simulink model "class_09"  (R2023b)
settings: Solver=VariableStepAuto  StartTime=0.0  StopTime=10.0  RelTol=1e-3
libraries: cstblocks x10
settings Model: Creator=klysm  LastModifiedBy=klysm

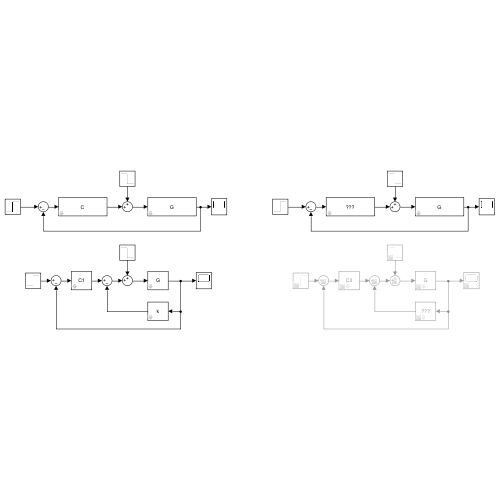
[thumbnail: Simulink's stored preview of the top-level diagram]
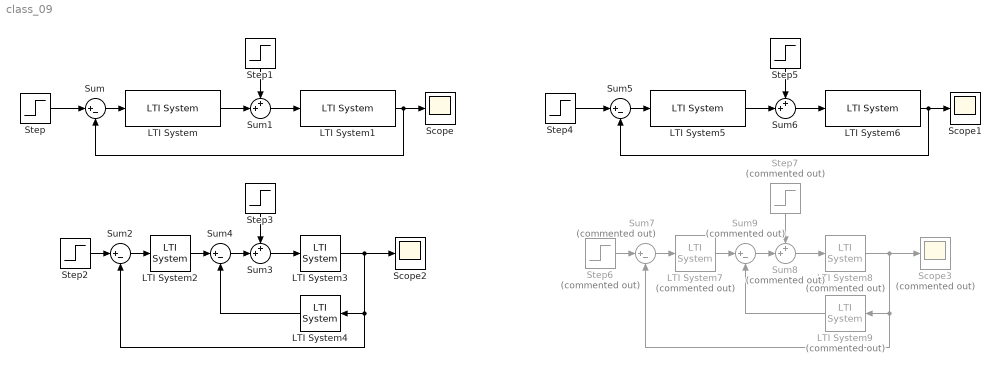
== system class_09 ==
  LTI System : cstblocks/LTI System  sys=C  IC=[]  PadeOrder=0
  LTI System1 : cstblocks/LTI System  sys=G  IC=[]  PadeOrder=0
  LTI System2 : cstblocks/LTI System  sys=C1  IC=[]  PadeOrder=0
  LTI System3 : cstblocks/LTI System  sys=G  IC=[]  PadeOrder=0
  LTI System4 : cstblocks/LTI System  sys=k  IC=[]  PadeOrder=0
  LTI System5 : cstblocks/LTI System  sys=C2  IC=[]  PadeOrder=0
  LTI System6 : cstblocks/LTI System  sys=G  IC=[]  PadeOrder=0
  LTI System7 : cstblocks/LTI System  Commented=on  sys=C3  IC=[]  PadeOrder=0
  LTI System8 : cstblocks/LTI System  Commented=on  sys=G  IC=[]  PadeOrder=0
  LTI System9 : cstblocks/LTI System  Commented=on  sys=C4  IC=[]  PadeOrder=0
  Scope : Scope
  Scope1 : Scope
  Scope2 : Scope
  Scope3 : Scope  Commented=on
  Step : Step  Time=0  SampleTime=0
  Step1 : Step  Time=5  After=-5  SampleTime=0
  Step2 : Step  Time=0  SampleTime=0
  Step3 : Step  Time=5  After=-5  SampleTime=0
  Step4 : Step  Time=0  SampleTime=0
  Step5 : Step  Time=5  After=-5  SampleTime=0
  Step6 : Step  Commented=on  Time=0  SampleTime=0
  Step7 : Step  Commented=on  Time=5  After=-5  SampleTime=0
  Sum{,2,4..5} (4 alike) : Sum  Inputs=|+-
  Sum1 : Sum  Inputs=++|
  Sum3 : Sum  Inputs=++|
  Sum6 : Sum  Inputs=++|
  Sum7 : Sum  Commented=on  Inputs=|+-
  Sum8 : Sum  Commented=on  Inputs=++|
  Sum9 : Sum  Commented=on  Inputs=|+-
  wires:
  LTI System/1 -> Sum1/2
  LTI System1/1 -> Sum/2, Scope/1
  Step/1 -> Sum/1
  Sum/1 -> LTI System/1
  Sum1/1 -> LTI System1/1
  Step1/1 -> Sum1/1
  Sum3/1 -> LTI System3/1
  Sum2/1 -> LTI System2/1
  Step3/1 -> Sum3/1
  LTI System3/1 -> Scope2/1, Sum2/2, LTI System4/1
  LTI System2/1 -> Sum4/1
  Step2/1 -> Sum2/1
  Sum4/1 -> Sum3/2
  LTI System4/1 -> Sum4/2
  Sum9/1 -> Sum8/2
  Step6/1 -> Sum7/1
  Sum7/1 -> LTI System7/1
  Step5/1 -> Sum6/1
  LTI System7/1 -> Sum9/1
  LTI System8/1 -> Scope3/1, Sum7/2, LTI System9/1
  LTI System9/1 -> Sum9/2
  Step4/1 -> Sum5/1
  LTI System6/1 -> Sum5/2, Scope1/1
  Step7/1 -> Sum8/1
  Sum8/1 -> LTI System8/1
  Sum6/1 -> LTI System6/1
  Sum5/1 -> LTI System5/1
  LTI System5/1 -> Sum6/2
